simulink model "modelref_robot_arm2_Model_Reference_Controller"  (R2014b)
settings: Solver=ode45  SolverMode=SingleTasking  StartTime=0.0  StopTime=60  RelTol=1e-3  AbsTol=1e-6
undefined symbols (not defined in the file): now, sfunxy2
settings Model: ExtModeTrigMode=oneshot  ExtModeArmWhenConnect=off  TunableVars=prueba  TunableVarsStorageClass=Auto  Creator=eyarrow  LastModifiedBy=david78k
settings DataIOCC: LimitDataPoints=off  SignalLoggingSaveFormat=ModelDataLogs  SaveOutput=off  SignalLoggingName=sigsOut
settings OptimizationCC: BooleanDataType=off  InlineParams=on  ExpressionDepthLimit=2147483647  InitFltsAndDblsToZero=on
settings DebuggingCC: SaveWithParameterizedLinksMsg=none  UnderspecifiedInitializationDetection=Classic  MergeDetectMultiDrivingBlocksExec=none  SignalResolutionControl=TryResolveAllWithWarning  SolverPrmCheckMsg=none  MultiTaskDSMMsg=warning  MultiTaskCondExecSysMsg=none  FcnCallInpInsideContextMsg=UseLocalSettings  StateNameClashWarn=warning  StrictBusMsg=None
settings HardwareCC: TargetUnknown=on
settings RTWCC: TemplateMakefile=grt_vc.tmf  IncludeERTFirstTime=on
settings GRTTargetCC: TargetFcnLib=ansi_tfl_tmw.mat  CombineOutputUpdateFcns=off  GRTInterface=on

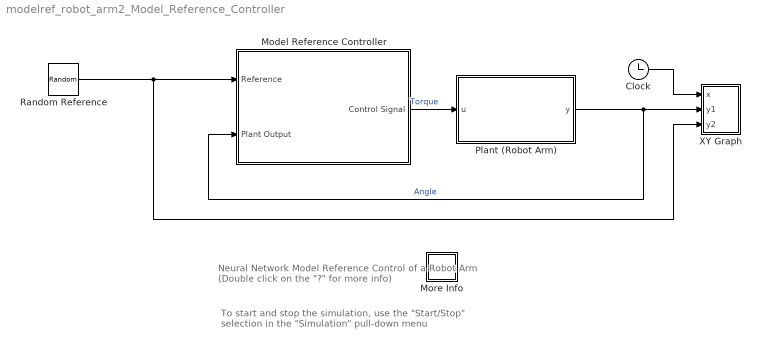
== system modelref_robot_arm2_Model_Reference_Controller ==
  note: Neural Network Model Reference Control of a Robot Arm
      | (Double click on the "?" for more info)
  note: To start and stop the simulation, use the "Start/Stop"
      | selection in the "Simulation" pull-down menu
  Clock : Clock
  Model Reference Controller : Subsystem  mask(NN Model Reference Control){Ts=0.05, S1=10, Ni=2, Nj=2, sim_file=robotarm, trainfun=trainlm, Use_validation=1, Use_Testing=1, Use_Inc_training=0, Use_previous_weights=1, max_i=15, min_i=-15, max_r=0.7, min_r=-0.7, sam_training=10000, sam_training_c=6000, epochs=300, epochs_c=10, minp=-14.988293499961703, maxp=14.923704088055537, mint=-3.3363903927128264, maxt=3.3206956917347106, Normalize=1, IW=[-0.011469687396173215 0.040727561644111239;1.075316793085894 3.6796838641403276;-1.0685679888493944 -1.4205632700292121;0.14367732817658238 0.6152803692703297;-0.46805195984615566 2.5890011355180014;-0.00099986462717487263 -0.0007252338745319933;0.020940253545379157 -0.065457349807555854;3.418928376293219 -2.1823823167283654;-0.0059345736730259191 -0.0070551937494547938;-2.1494988517134881 -2.6774267562058767], LW1_2=[-1.3659168016442902 3.6192798596548861;5.3731109044400727 0.69786952127836066;1.4450743609809416 -1.9984706683615918;2.5525543014913454 -1.4826245221004251;3.4559923743807279 -2.3555418718376742;-0.35124450033305005 0.17636235061342501;4.2690027031324904 -4.7193108091953446;-3.6662434033635201 3.7972392042066518;-1.9187608842814841 0.75056361802973048;4.6610943267477873 1.5166165956758935], LW2_1=[0.013403472002469021 -2.3473487105238961e-005 7.2702651156598242e-005 0.0013482923593579168 -0.00016616129434688127 -5.8011812414478516 -0.010014055898134575 3.8530349704142433e-005 -0.19642052374504862 0.00010666269673941641], B1=[-1.5792545839864678;-1.1799157268366136;0.14188462146879066;-0.17920873848457491;-0.41999647602943724;0.34136385139415004;-0.37981883756521306;3.4871946858243157;-1.2726850310343014;5.4629125163629446], B2=1.7477024054779804, S1c=13, Limit_output=1, min_output=-3.1, max_output=3.1, Ref_file=robotref, Nrc=2, Nic=1, Njc=2, IW_y=[-0.28830069175292433 -0.40646751091557659;0.28595139003619108 -0.57417214335064837;0.1336707314980988 -0.093036501318070008;-0.2019599111771567 -0.025678078476613929;0.84713300279901316 0.72007254571163293;0.36748636396046436 1.0000215468311262;0.066756131692085038 0.38725405501697979;-0.17019741781512493 0.5165521764796247;0.46609436858091502 0.6239894923394288;0.46324541261221525 0.086935183955805476;-0.44961103869309321 0.25383246728779613;-0.048218807870090009 -0.39894955367872065;-0.61986971529707569 0.058497236367605482], IW_u=[-0.07687034475824113;-0.040567981957116965;-0.25789970936411499;-0.018721032897876001;0.028817060765054997;-0.31264836826089376;0.18921583903705724;-0.61261686016868233;-0.16307742563522379;-0.074462566067034761;0.056746504440949669;0.21187656712469111;-0.056770151099039622], IW_r=[-1.0362660354173303 1.4688605237132542;0.42403471351339406 0.09884618409637784;1.4428485632037449 2.6760930779748908;1.8930687109886244 -1.6745583333584542;1.065008106228545 -0.87008906986887113;-1.7918541807535311 1.0744242311327989;1.7753415232484064 1.3072326174145978;1.5573152998068889 -0.888848087048283;-1.2394371299457376 1.3050943120462382;1.0278618084899167 -0.18597892573437988;-1.0916083269493662 1.9125168626791282;0.99122416074121877 -0.14414702314486633;0.95925862503152526 -0.61012901799671015], B1_c=[2.306994450802522;-1.9000153414921086;-1.3008630649724051;1.258877310519851;-0.12980477297087051;0.12368183073014268;-0.85644903109457482;-0.41889440632432878;0.98725693995885255;1.1772875199263355;-1.6349473404405293;2.0825629905810632;-2.3440725161816367], B2_c=0.82217357531165991, LW_c=[-0.55529719028462121 -0.31761057023184625 -0.015052391499648663 0.30814748264618441 0.98893787454368642 0.37299266080087584 0.016791395741317917 0.40413014544500553 -0.069013433882631259 0.18826999272001291 -0.21076173160301825 -0.64099798332438396 0.28967605954116094], retraining_c=5, max_i_int=2, min_i_int=0.1, max_r_int=2, min_r_int=0.1}
      mask prompts: Ts "Sample time"; trainfun "Training function Identification"; Limit_output "Limit output"
      mask help: Neural network model reference controller. You first train a neural network model of the plant to be controlled. Then train the controller so that the plant output will follow the output of a reference model. Double-click the Model Reference Control block to begin the plant and controller training.
      mask init:
      | xl = [0   .53     .53     .92   .92   .53   .53  NaN ];
      | yl = [.95 .95 1.05 1.05 .3   .3   .95 NaN  ];
      | x2 = [0 .53    NaN .92 1.2  ];
      | y2 = [.39 .39   NaN .65 .65  ];
      | t=(0:24)/24*2*pi;
      | xs = .07*cos(t)+.9;
      | ys = .07*sin(t)+.75;
      | 
      | x1t=.03; y1t=.31;
      | x2t=.03; y2t=.8;
      | x3t=.77; y3t=.53;
      | x4t=.77; y4t=.44;
      | x5t=.45; y5t=.66;
      | x6t=.45; y6t=.55;
      | x7t=.45; y7t=.44;
      settings: OpenFcn=nncontrolutil('nnmodref','',gcbh,gcb,'');
      mask TypeOptions trainfun: trainbfg | trainbr  | traincgb | traincgf | traincgp | traingd | traingdm | traingda | traingdx | trainlm  | trainoss | trainrp  | trainscg
      mask Display:
      | plot([[xl NaN x2]*.9-.075 ], [[yl  NaN y2]*.9-.1 ]);
      | text(x1t,y1t,'Plant Output');
      | text(x2t,y2t,'Reference');
      | text(x3t,y3t,'Control');
      | text(x4t,y4t,'Signal');
      | text(x5t,y5t,'Neural');
      | text(x6t,y6t,'Network');
      | text(x7t,y7t,'Controller');
  More Info : Subsystem
      mask Display: disp('?')
  Plant (Robot Arm) : Subsystem
      mask Display: plot([-10],[0],[10],[0],[-2 -2 2 2 -2],[5 4 4 5 5],[0 3],[4.5 0.5])
  Random Reference : UniformRandomNumber  Minimum=-0.5  Maximum=0.5  Seed=round(now)  SampleTime=10
  XY Graph : Subsystem  LoadFcn=sfunxy2([],[],[],'LoadBlock')  StartFcn=sfunxy2([],[],[],'Start')  StopFcn=sfunxy2([],[],[],'Stop')  mask(XY scope.){xmin=0, xmax=5, ymin=-1, ymax=1, st=-1}
      mask prompts: xmin "x-min:"; xmax "x-max:"; ymin "y-min:"; ymax "y-max:"; st "Sample time:"
      mask help: XY scope using MATLAB graph window. First input is used as time base. Enter plotting ranges.
      settings: CopyFcn=sfunxy2([],[],[],'CopyBlock')  DeleteFcn=sfunxy2([],[],[],'DeleteBlock')  NameChangeFcn=sfunxy2([],[],[],'NameChange')
      mask Help: This block can be used to explore limit cycles. Look at the function sfunxy.m to see how it works.
      mask Display: plot([.05 .95 .95 .05 .05],[.45 .45 .95 .95 .45], 0.5+cos(0:0.1:2*pi)*0.3,0.7+sin(0:0.1:2*pi)*0.2)
  wires:
  Plant (Robot Arm)/1(y) -> XY Graph/2(y1), Model Reference Controller/2(Plant Output)  "Angle"
  Model Reference Controller/1(Control Signal) -> Plant (Robot Arm)/1(u)  "Torque"
  Clock/1 -> XY Graph/1(x)
  Random Reference/1 -> Model Reference Controller/1(Reference), XY Graph/3(y2)

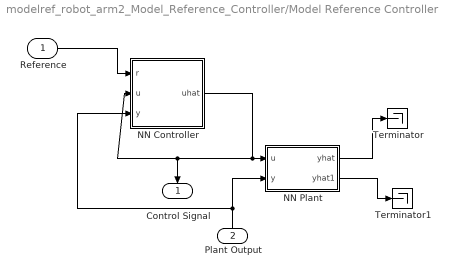
== system modelref_robot_arm2_Model_Reference_Controller/Model Reference Controller ==
  Reference : Inport
  Plant Output : Inport  Port=2
  NN Controller : Subsystem
  NN Plant : Subsystem
  Terminator : Terminator
  Terminator1 : Terminator
  Control Signal : Outport
  wires:
  Plant Output/1 -> NN Plant/2(y), NN Controller/3(y)
  NN Controller/1(uhat) -> NN Plant/1(u), Control Signal/1, NN Controller/2(u)
  Reference/1 -> NN Controller/1(r)
  NN Plant/1(yhat) -> Terminator/1
  NN Plant/2(yhat1) -> Terminator1/1

== system modelref_robot_arm2_Model_Reference_Controller/More Info ==
  note: This system simulates model reference control
      | of a single-link robot arm.
  note: Double-click on the Model Reference Controller block
      | to train the neural network controller and plant model.
  note: For more information on what the controller
      | does, look under the mask of the Model Reference
      | Controller block.

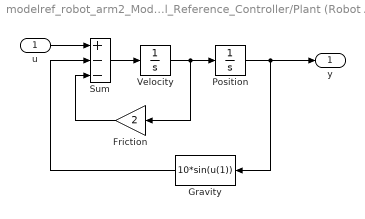
== system modelref_robot_arm2_Model_Reference_Controller/Plant (Robot Arm) ==
  u : Inport
  Friction : Gain  Gain=2  SaturateOnIntegerOverflow=on  OutDataTypeStr=Inherit: Same as input  ParamDataTypeStr=Inherit: Same as input
  Gravity : Fcn  Expr=10*sin(u(1))
  Position : Integrator
  Sum : Sum  Inputs=+--  SaturateOnIntegerOverflow=on  InputSameDT=on  OutDataTypeStr=Inherit: Same as first input
  Velocity : Integrator
  y : Outport
  wires:
  Position/1 -> y/1, Gravity/1
  u/1 -> Sum/1
  Sum/1 -> Velocity/1
  Gravity/1 -> Sum/2
  Velocity/1 -> Position/1, Friction/1
  Friction/1 -> Sum/3

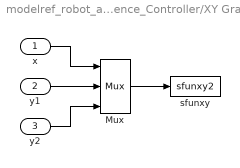
== system modelref_robot_arm2_Model_Reference_Controller/XY Graph ==
  x : Inport
  y1 : Inport  Port=2
  y2 : Inport  Port=3
  Mux : Mux  Inputs=3
  sfunxy : S-Function  FunctionName=sfunxy2  Parameters=[xmin xmax ymin ymax], st  EnableBusSupport=off
  wires:
  Mux/1 -> sfunxy/1
  x/1 -> Mux/1
  y1/1 -> Mux/2
  y2/1 -> Mux/3

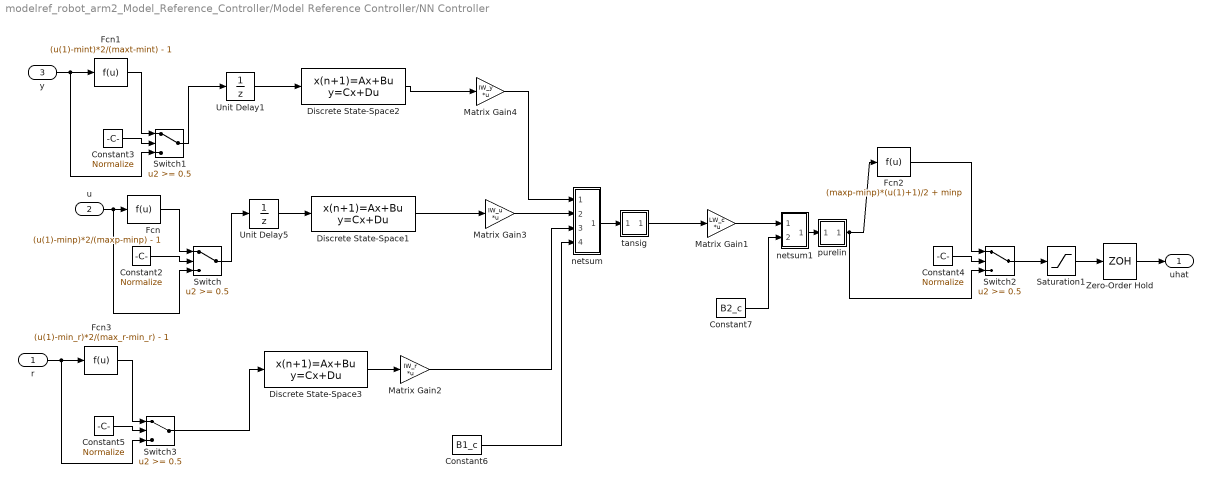
== system modelref_robot_arm2_Model_Reference_Controller/Model Reference Controller/NN Controller ==
  r : Inport
  u : Inport  Port=2
  y : Inport  Port=3
  Constant{2..5} (4 alike) : Constant  Value=Normalize
  Constant6 : Constant  Value=B1_c
  Constant7 : Constant  Value=B2_c
  Discrete State-Space1 : DiscreteStateSpace  A=[zeros(1,max([Nic-1 1]));eye(Nic-2,Nic-1)]  B=eye(max([Nic-1 1]),1)  C=[zeros(1,max([Nic-1 1]));eye(Nic-1,Nic-1)]  D=eye(Nic,1)  SampleTime=Ts
  Discrete State-Space2 : DiscreteStateSpace  A=[zeros(1,max([Njc-1 1]));eye(Njc-2,Njc-1)]  B=eye(max([Njc-1 1]),1)  C=[zeros(1,max([Njc-1 1]));eye(Njc-1,Njc-1)]  D=eye(Njc,1)  SampleTime=Ts
  Discrete State-Space3 : DiscreteStateSpace  A=[zeros(1,max([Nrc-1 1]));eye(Nrc-2,Nrc-1)]  B=eye(max([Nrc-1 1]),1)  C=[zeros(1,max([Nrc-1 1]));eye(Nrc-1,Nrc-1)]  D=eye(Nrc,1)  SampleTime=Ts
  Fcn : Fcn  Expr=(u(1)-minp)*2/(maxp-minp) - 1
  Fcn1 : Fcn  Expr=(u(1)-mint)*2/(maxt-mint) - 1
  Fcn2 : Fcn  Expr=(maxp-minp)*(u(1)+1)/2 + minp
  Fcn3 : Fcn  Expr=(u(1)-min_r)*2/(max_r-min_r) - 1
  Matrix Gain1 : Gain  Gain=LW_c  Multiplication=Matrix(K*u)  SaturateOnIntegerOverflow=on  OutDataTypeStr=Inherit: Same as input  ParamDataTypeStr=Inherit: Same as input
  Matrix Gain2 : Gain  Gain=IW_r  Multiplication=Matrix(K*u)  SaturateOnIntegerOverflow=on  OutDataTypeStr=Inherit: Same as input  ParamDataTypeStr=Inherit: Same as input
  Matrix Gain3 : Gain  Gain=IW_u  Multiplication=Matrix(K*u)  SaturateOnIntegerOverflow=on  OutDataTypeStr=Inherit: Same as input  ParamDataTypeStr=Inherit: Same as input
  Matrix Gain4 : Gain  Gain=IW_y  Multiplication=Matrix(K*u)  SaturateOnIntegerOverflow=on  OutDataTypeStr=Inherit: Same as input  ParamDataTypeStr=Inherit: Same as input
  Saturation1 : Saturate  UpperLimit=max_i  LowerLimit=min_i
  Switch{,1..3} (4 alike) : Switch  Threshold=0.5  SaturateOnIntegerOverflow=on  InputSameDT=on
  Unit Delay1 : UnitDelay  SampleTime=Ts
  Unit Delay5 : UnitDelay  SampleTime=Ts
  Zero-Order Hold : ZeroOrderHold  SampleTime=Ts
  netsum : Subsystem
      mask Display: disp('+')
  netsum1 : Subsystem
      mask Display: disp('+')
  purelin : Subsystem
      mask Display: plot([-1 1],[0 0],[-1 1],[-1 1])
  tansig : Subsystem
      mask Display: plot([-1 1],[0 0],[-1 -.9 -.8 -.7 -.6 -.5 -.4 -.3 -.2 -.1 0 .1 .2 .3 .4 .5 .6 .7 .8 .9 1],2./(1+exp(-8*[-1 -.9 -.8 -.7 -.6 -.5 -.4 -.3 -.2 -.1 0 .1 .2 .3 .4 .5 .6 .7 .8 .9 1]))-1)
  uhat : Outport
  wires:
  Matrix Gain4/1 -> netsum/1(In1)
  Matrix Gain3/1 -> netsum/2(In2)
  Constant6/1 -> netsum/4(In4)
  Switch/1 -> Unit Delay5/1
  u/1 -> Switch/3, Fcn/1
  Constant2/1 -> Switch/2
  Constant3/1 -> Switch1/2
  Switch1/1 -> Unit Delay1/1
  Fcn1/1 -> Switch1/1
  y/1 -> Fcn1/1, Switch1/3
  Constant5/1 -> Switch3/2
  Fcn3/1 -> Switch3/1
  r/1 -> Fcn3/1, Switch3/3
  netsum/1(Out1) -> tansig/1(n)
  Matrix Gain2/1 -> netsum/3(In3)
  netsum1/1(Out1) -> purelin/1(n)
  Matrix Gain1/1 -> netsum1/1(In1)
  Constant4/1 -> Switch2/2
  purelin/1(a) -> Switch2/3, Fcn2/1
  Switch2/1 -> Saturation1/1
  Constant7/1 -> netsum1/2(In2)
  Discrete State-Space3/1 -> Matrix Gain2/1
  Zero-Order Hold/1 -> uhat/1
  Saturation1/1 -> Zero-Order Hold/1
  Unit Delay5/1 -> Discrete State-Space1/1
  Unit Delay1/1 -> Discrete State-Space2/1
  Switch3/1 -> Discrete State-Space3/1
  Discrete State-Space2/1 -> Matrix Gain4/1
  tansig/1(a) -> Matrix Gain1/1
  Discrete State-Space1/1 -> Matrix Gain3/1
  Fcn/1 -> Switch/1
  Fcn2/1 -> Switch2/1

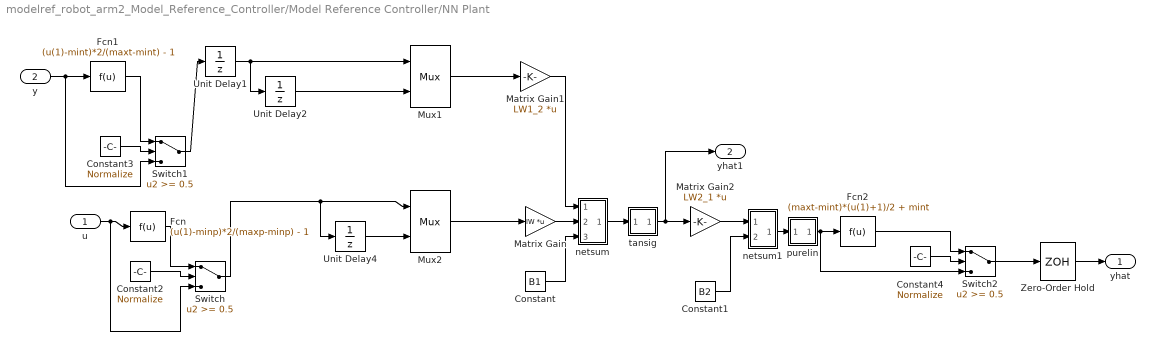
== system modelref_robot_arm2_Model_Reference_Controller/Model Reference Controller/NN Plant ==
  u : Inport
  y : Inport  Port=2
  Constant : Constant  Value=B1
  Constant1 : Constant  Value=B2
  Constant2 : Constant  Value=Normalize
  Constant3 : Constant  Value=Normalize
  Constant4 : Constant  Value=Normalize
  Fcn : Fcn  Expr=(u(1)-minp)*2/(maxp-minp) - 1
  Fcn1 : Fcn  Expr=(u(1)-mint)*2/(maxt-mint) - 1
  Fcn2 : Fcn  Expr=(maxt-mint)*(u(1)+1)/2 + mint
  Matrix Gain : Gain  Gain=IW  Multiplication=Matrix(K*u)  SaturateOnIntegerOverflow=on  OutDataTypeStr=Inherit: Same as input  ParamDataTypeStr=Inherit: Same as input
  Matrix Gain1 : Gain  Gain=LW1_2  Multiplication=Matrix(K*u)  SaturateOnIntegerOverflow=on  OutDataTypeStr=Inherit: Same as input  ParamDataTypeStr=Inherit: Same as input
  Matrix Gain2 : Gain  Gain=LW2_1  Multiplication=Matrix(K*u)  SaturateOnIntegerOverflow=on  OutDataTypeStr=Inherit: Same as input  ParamDataTypeStr=Inherit: Same as input
  Mux1 : Mux  Inputs=2
      settings: DisplayOption=signals
  Mux2 : Mux  Inputs=2
      settings: DisplayOption=signals
  Switch : Switch  Threshold=0.5  SaturateOnIntegerOverflow=on  InputSameDT=on
  Switch1 : Switch  Threshold=0.5  SaturateOnIntegerOverflow=on  InputSameDT=on
  Switch2 : Switch  Threshold=0.5  SaturateOnIntegerOverflow=on  InputSameDT=on
  Unit Delay1 : UnitDelay  SampleTime=Ts
  Unit Delay2 : UnitDelay  SampleTime=Ts
  Unit Delay4 : UnitDelay  SampleTime=Ts
  Zero-Order Hold : ZeroOrderHold  SampleTime=Ts
  netsum : Subsystem
      mask Display: disp('+')
  netsum1 : Subsystem
      mask Display: disp('+')
  purelin : Subsystem
      mask Display: plot([-1 1],[0 0],[-1 1],[-1 1])
  tansig : Subsystem
      mask Display: plot([-1 1],[0 0],[-1 -.9 -.8 -.7 -.6 -.5 -.4 -.3 -.2 -.1 0 .1 .2 .3 .4 .5 .6 .7 .8 .9 1],2./(1+exp(-8*[-1 -.9 -.8 -.7 -.6 -.5 -.4 -.3 -.2 -.1 0 .1 .2 .3 .4 .5 .6 .7 .8 .9 1]))-1)
  yhat : Outport
  yhat1 : Outport  Port=2
  wires:
  netsum1/1(Out1) -> purelin/1(n)
  Constant1/1 -> netsum1/2(In2)
  Matrix Gain2/1 -> netsum1/1(In1)
  netsum/1(Out1) -> tansig/1(n)
  Constant/1 -> netsum/3(In3)
  Matrix Gain1/1 -> netsum/1(In1)
  Matrix Gain/1 -> netsum/2(In2)
  tansig/1(a) -> Matrix Gain2/1, yhat1/1
  Constant4/1 -> Switch2/2
  Fcn2/1 -> Switch2/1
  purelin/1(a) -> Fcn2/1, Switch2/3
  Mux2/1 -> Matrix Gain/1
  Fcn/1 -> Switch/1
  u/1 -> Fcn/1, Switch/3
  Constant2/1 -> Switch/2
  Mux1/1 -> Matrix Gain1/1
  Constant3/1 -> Switch1/2
  Switch1/1 -> Unit Delay1/1
  Fcn1/1 -> Switch1/1
  y/1 -> Fcn1/1, Switch1/3
  Unit Delay1/1 -> Mux1/1, Unit Delay2/1
  Unit Delay2/1 -> Mux1/2
  Unit Delay4/1 -> Mux2/2
  Switch/1 -> Mux2/1, Unit Delay4/1
  Zero-Order Hold/1 -> yhat/1
  Switch2/1 -> Zero-Order Hold/1

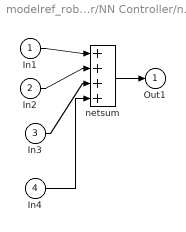
== system modelref_robot_arm2_Model_Reference_Controller/Model Reference Controller/NN Controller/netsum ==
  In1 : Inport
  In2 : Inport  Port=2
  In3 : Inport  Port=3
  In4 : Inport  Port=4
  netsum : Sum  Inputs=4  SaturateOnIntegerOverflow=on  InputSameDT=on  OutDataTypeStr=Inherit: Same as first input
  Out1 : Outport
  wires:
  In1/1 -> netsum/1
  In2/1 -> netsum/2
  netsum/1 -> Out1/1
  In3/1 -> netsum/3
  In4/1 -> netsum/4

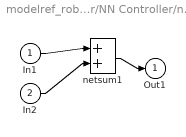
== system modelref_robot_arm2_Model_Reference_Controller/Model Reference Controller/NN Controller/netsum1 ==
  In1 : Inport
  In2 : Inport  Port=2
  netsum1 : Sum  Inputs=2  SaturateOnIntegerOverflow=on  InputSameDT=on  OutDataTypeStr=Inherit: Same as first input
  Out1 : Outport
  wires:
  In1/1 -> netsum1/1
  In2/1 -> netsum1/2
  netsum1/1 -> Out1/1

== system modelref_robot_arm2_Model_Reference_Controller/Model Reference Controller/NN Controller/purelin ==
  n : Inport
  a : Outport
  wires:
  n/1 -> a/1

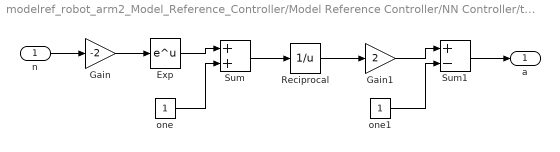
== system modelref_robot_arm2_Model_Reference_Controller/Model Reference Controller/NN Controller/tansig ==
  n : Inport
  Exp : Math  SaturateOnIntegerOverflow=on
  Gain : Gain  Gain=-2  SaturateOnIntegerOverflow=on  OutDataTypeStr=Inherit: Same as input  ParamDataTypeStr=Inherit: Same as input
  Gain1 : Gain  Gain=2  SaturateOnIntegerOverflow=on  OutDataTypeStr=Inherit: Same as input  ParamDataTypeStr=Inherit: Same as input
  Reciprocal : Math  Operator=reciprocal  SaturateOnIntegerOverflow=on
  Sum : Sum  SaturateOnIntegerOverflow=on  InputSameDT=on  OutDataTypeStr=Inherit: Same as first input
  Sum1 : Sum  Inputs=+-  SaturateOnIntegerOverflow=on  InputSameDT=on  OutDataTypeStr=Inherit: Same as first input
  one : Constant
  one1 : Constant
  a : Outport
  wires:
  n/1 -> Gain/1
  Gain/1 -> Exp/1
  Exp/1 -> Sum/1
  one/1 -> Sum/2
  Sum/1 -> Reciprocal/1
  Reciprocal/1 -> Gain1/1
  Gain1/1 -> Sum1/1
  one1/1 -> Sum1/2
  Sum1/1 -> a/1

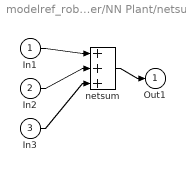
== system modelref_robot_arm2_Model_Reference_Controller/Model Reference Controller/NN Plant/netsum ==
  In1 : Inport
  In2 : Inport  Port=2
  In3 : Inport  Port=3
  netsum : Sum  Inputs=3  SaturateOnIntegerOverflow=on  InputSameDT=on  OutDataTypeStr=Inherit: Same as first input
  Out1 : Outport
  wires:
  In1/1 -> netsum/1
  In2/1 -> netsum/2
  In3/1 -> netsum/3
  netsum/1 -> Out1/1

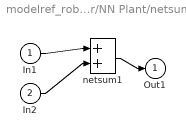
== system modelref_robot_arm2_Model_Reference_Controller/Model Reference Controller/NN Plant/netsum1 ==
  In1 : Inport
  In2 : Inport  Port=2
  netsum1 : Sum  Inputs=2  SaturateOnIntegerOverflow=on  InputSameDT=on  OutDataTypeStr=Inherit: Same as first input
  Out1 : Outport
  wires:
  In1/1 -> netsum1/1
  In2/1 -> netsum1/2
  netsum1/1 -> Out1/1

== system modelref_robot_arm2_Model_Reference_Controller/Model Reference Controller/NN Plant/purelin ==
  n : Inport
  a : Outport
  wires:
  n/1 -> a/1

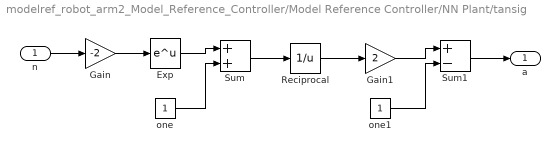
== system modelref_robot_arm2_Model_Reference_Controller/Model Reference Controller/NN Plant/tansig ==
  n : Inport
  Exp : Math  SaturateOnIntegerOverflow=on
  Gain : Gain  Gain=-2  SaturateOnIntegerOverflow=on  OutDataTypeStr=Inherit: Same as input  ParamDataTypeStr=Inherit: Same as input
  Gain1 : Gain  Gain=2  SaturateOnIntegerOverflow=on  OutDataTypeStr=Inherit: Same as input  ParamDataTypeStr=Inherit: Same as input
  Reciprocal : Math  Operator=reciprocal  SaturateOnIntegerOverflow=on
  Sum : Sum  SaturateOnIntegerOverflow=on  InputSameDT=on  OutDataTypeStr=Inherit: Same as first input
  Sum1 : Sum  Inputs=+-  SaturateOnIntegerOverflow=on  InputSameDT=on  OutDataTypeStr=Inherit: Same as first input
  one : Constant
  one1 : Constant
  a : Outport
  wires:
  n/1 -> Gain/1
  Gain/1 -> Exp/1
  Exp/1 -> Sum/1
  one/1 -> Sum/2
  Sum/1 -> Reciprocal/1
  Reciprocal/1 -> Gain1/1
  Gain1/1 -> Sum1/1
  one1/1 -> Sum1/2
  Sum1/1 -> a/1
